simulink library "csc_ltg_landing_terminal_guidance_lib"  (R2015b)
settings: Solver=ode45  StartTime=0.0  StopTime=10.0  RelTol=1e-3
values from neighbouring files (symbols this model uses):
  gdn_altitude_transition_free_drift_landing = 1.00    (= 1)    [csc_gal_gdn_approach_landing_init.m]
  gdn_altitude_transition_free_drift_takeoff = -1.0    (= -1)    [csc_gal_gdn_approach_landing_init.m]
undefined symbols (not defined in the file or in its folder): gal_grav_surface_topo
libraries: util_info_lib x1, csc_tlt_takeoff_landing_table_guidance_lib x1, csu_pwm_pwpf_logic_lib x1, util_extra_lib x1
settings Model: Creator=escrane  LastModifiedBy=jimkaidy
settings DataIOCC: SaveFormat=Array
settings DebuggingCC: UnderspecifiedInitializationDetection=Classic  MergeDetectMultiDrivingBlocksExec=none  SolverPrmCheckMsg=warning
settings HardwareCC: ProdBitPerPointer=32  ProdLargestAtomicFloat=None  ProdIntDivRoundTo=Undefined  ProdEndianess=Unspecified  ProdWordSize=32  ProdHWDeviceType=32-bit Generic
settings GRTTargetCC: GeneratePreprocessorConditionals=Disable all
settings ConfigComp: CovModelRefEnable=Off  CovSFcnEnable=off

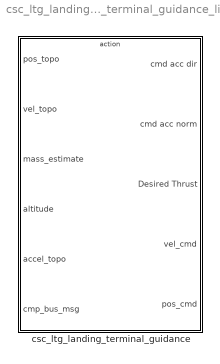
== system csc_ltg_landing_terminal_guidance_lib ==
  csc_ltg_landing_terminal_guidance : Subsystem  TreatAsAtomicUnit=on

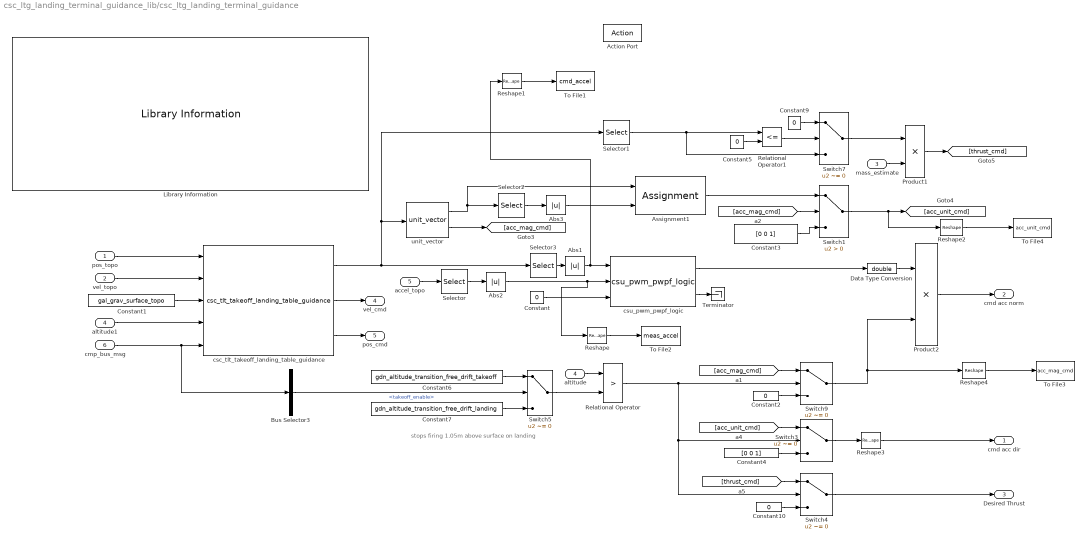
== system csc_ltg_landing_terminal_guidance_lib/csc_ltg_landing_terminal_guidance ==
  note: stops firing 1.05m above surface on landing
  pos_topo : Inport
  vel_topo : Inport  Port=2
  mass_estimate : Inport  Port=3
  altitude : Inport  Port=4
  accel_topo : Inport  Port=5
  cmp_bus_msg : Inport  Port=6
  Action Port : ActionPort
  Abs1 : Abs
  Abs2 : Abs
  Abs3 : Abs
  Assignment1 : Assignment  IndexOptions=Index vector (dialog)  Indices=3  OutputSizes=1
  Bus Selector3 : BusSelector  OutputSignals=takeoff_enable
  Constant{,2,5,9} (4 alike) : Constant  Value=0
  Constant1 : Constant  Value=gal_grav_surface_topo
  Constant10 : Constant  Value=0  OutDataTypeStr=uint8
  Constant3 : Constant  Value=[0 0 1]
  Constant4 : Constant  Value=[0 0 1]
  Constant6 : Constant  Value=gdn_altitude_transition_free_drift_takeoff  VectorParams1D=off
  Constant7 : Constant  Value=gdn_altitude_transition_free_drift_landing  VectorParams1D=off
  Data Type Conversion : DataTypeConversion  OutDataTypeStr=double
  Library Information : util_info_lib/Library Information  owner='NONE'
  Product1 : Product
  Product2 : Product  RndMeth=Zero
  Relational Operator : RelationalOperator  Operator=>  OutDataTypeStr=boolean
  Relational Operator1 : RelationalOperator  Operator=<=  OutDataTypeStr=boolean
  Reshape{,1..4} (5 alike) : Reshape
  Selector{,1..3} (4 alike) : Selector  InputPortWidth=3  IndexOptions=Index vector (dialog)  Indices=[3]  OutputSizes=1
  Switch1 : Switch  Criteria=u2 > Threshold
  Switch{3..5,7,9} (5 alike) : Switch  Criteria=u2 ~= 0
  Terminator : Terminator
  To File1 : ToFile  Filename=cmd_accel  MatrixName=cmd_accel  SaveFormat=Timeseries
  To File2 : ToFile  Filename=meas_accel  MatrixName=meas_accel  SaveFormat=Timeseries
  To File3 : ToFile  Filename=acc_mag_cmd  MatrixName=acc_mag_cmd  SaveFormat=Timeseries
  To File4 : ToFile  Filename=acc_unit_cmd  MatrixName=acc_unit_cmd  SaveFormat=Timeseries
  altitude1 : InportShadow  Port=4
  csc_tlt_takeoff_landing_table_guidance : csc_tlt_takeoff_landing_table_guidance_lib/csc_tlt_takeoff_landing_table_guidance  VariantControl=(default)
  csu_pwm_pwpf_logic : csu_pwm_pwpf_logic_lib/csu_pwm_pwpf_logic  Km=ltg_pwpf_accel_err_km  Tm=ltg_pwpf_accel_integ_tm  dt=-1  trigger_on=ltg_pwpf_trigger_on_alpha  trigger_off=ltg_pwpf_trigger_off_alpha
  unit_vector : util_extra_lib/unit_vector  SystemSampleTime=-1
  cmd acc dir : Outport  InitialOutput=[0 0 1]'
  cmd acc norm : Outport  Port=2  InitialOutput=0
  Desired Thrust : Outport  Port=3  InitialOutput=0
  vel_cmd : Outport  Port=4  InitialOutput=0
  pos_cmd : Outport  Port=5  InitialOutput=0
  wires:
  csc_tlt_takeoff_landing_table_guidance/3 -> pos_cmd/1
  csc_tlt_takeoff_landing_table_guidance/2 -> vel_cmd/1
  csc_tlt_takeoff_landing_table_guidance/1 -> unit_vector/1, Selector1/1, Selector3/1
  Assignment1/1 -> Switch1/1
  [acc_mag_cmd] -> Switch1/2
  Selector1/1 -> Switch7/3, Relational Operator1/1
  Constant5/1 -> Relational Operator1/2
  Product2/1 -> cmd acc norm/1
  Data Type Conversion/1 -> Product2/1
  csu_pwm_pwpf_logic/2 -> Terminator/1
  accel_topo/1 -> Selector/1
  Abs1/1 -> Reshape1/1, csu_pwm_pwpf_logic/1
  Abs2/1 -> Reshape/1, csu_pwm_pwpf_logic/2
  Selector3/1 -> Abs1/1
  Selector/1 -> Abs2/1
  Constant/1 -> csu_pwm_pwpf_logic/3
  altitude1/1 -> csc_tlt_takeoff_landing_table_guidance/4
  Reshape3/1 -> cmd acc dir/1
  vel_topo/1 -> csc_tlt_takeoff_landing_table_guidance/2
  pos_topo/1 -> csc_tlt_takeoff_landing_table_guidance/1
  Constant1/1 -> csc_tlt_takeoff_landing_table_guidance/3
  cmp_bus_msg/1 -> Bus Selector3/1, csc_tlt_takeoff_landing_table_guidance/5
  Switch4/1 -> Desired Thrust/1
  Constant10/1 -> Switch4/3
  [thrust_cmd] -> Switch4/1
  Product1/1 -> [thrust_cmd]
  altitude/1 -> Relational Operator/1
  Switch7/1 -> Product1/1
  Relational Operator1/1 -> Switch7/2
  Constant9/1 -> Switch7/1
  mass_estimate/1 -> Product1/2
  Switch3/1 -> Reshape3/1
  Relational Operator/1 -> Switch9/2, Switch3/2, Switch4/2
  unit_vector/2 -> [acc_mag_cmd]
  unit_vector/1 -> Assignment1/1, Selector2/1
  [acc_unit_cmd] -> Switch3/1
  [acc_mag_cmd] -> Switch9/1
  Constant2/1 -> Switch9/3
  Constant4/1 -> Switch3/3
  Bus Selector3/1 -> Switch5/2  "<takeoff_enable>"
  Constant7/1 -> Switch5/3
  Constant6/1 -> Switch5/1
  Switch5/1 -> Relational Operator/2
  Selector2/1 -> Abs3/1
  Abs3/1 -> Assignment1/2
  Reshape/1 -> To File2/1
  Reshape1/1 -> To File1/1
  Reshape4/1 -> To File3/1
  Switch1/1 -> Reshape2/1, [acc_unit_cmd]
  Reshape2/1 -> To File4/1
  Constant3/1 -> Switch1/3
  Switch9/1 -> Reshape4/1, Product2/2
  csu_pwm_pwpf_logic/1 -> Data Type Conversion/1
